simulink model "tle2eci_test"  (R2016b)
settings: Solver=VariableStepAuto  StartTime=0.0  StopTime=10.0  RelTol=1e-3
undefined symbols (not defined in the file or in its folder): fsw_params
libraries: GPS_time_lib x1, sgp4_lib_fsw x1, time_coord_rotation_lib x1, tle2eci_coarse_lib x1
settings Model: Creator=Taylor  LastModifiedBy=Taylor

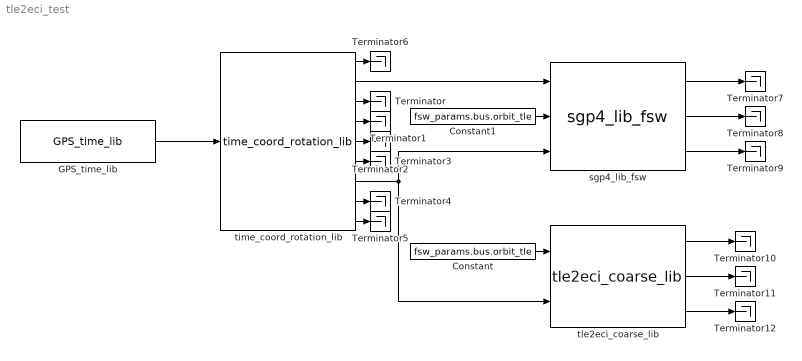
== system tle2eci_test ==
  Constant : Constant  Value=fsw_params.bus.orbit_tle
  Constant1 : Constant  Value=fsw_params.bus.orbit_tle
  GPS_time_lib : GPS_time_lib/GPS_time_lib
  Terminator{,1..12} (13 alike) : Terminator
  sgp4_lib_fsw : sgp4_lib_fsw/sgp4_lib_fsw
  time_coord_rotation_lib : time_coord_rotation_lib/time_coord_rotation_lib
  tle2eci_coarse_lib : tle2eci_coarse_lib/tle2eci_coarse_lib
  wires:
  GPS_time_lib/1 -> time_coord_rotation_lib/1
  time_coord_rotation_lib/7 -> tle2eci_coarse_lib/2, sgp4_lib_fsw/3
  time_coord_rotation_lib/2 -> sgp4_lib_fsw/1
  Constant/1 -> tle2eci_coarse_lib/1
  Constant1/1 -> sgp4_lib_fsw/2
  time_coord_rotation_lib/1 -> Terminator6/1
  time_coord_rotation_lib/3 -> Terminator/1
  time_coord_rotation_lib/4 -> Terminator1/1
  time_coord_rotation_lib/5 -> Terminator2/1
  time_coord_rotation_lib/6 -> Terminator3/1
  time_coord_rotation_lib/8 -> Terminator4/1
  time_coord_rotation_lib/9 -> Terminator5/1
  sgp4_lib_fsw/1 -> Terminator7/1
  sgp4_lib_fsw/3 -> Terminator9/1
  sgp4_lib_fsw/2 -> Terminator8/1
  tle2eci_coarse_lib/1 -> Terminator10/1
  tle2eci_coarse_lib/2 -> Terminator11/1
  tle2eci_coarse_lib/3 -> Terminator12/1
